simulink model "Balloon_Animation"  (R2020a)
settings: Solver=VariableStepAuto  StartTime=0.0  StopTime=100  RelTol=1e-3
libraries: vrlib x3, simulink x2, visionsinks x1
settings Model: Creator=Jeffrey  LastModifiedBy=seanchai

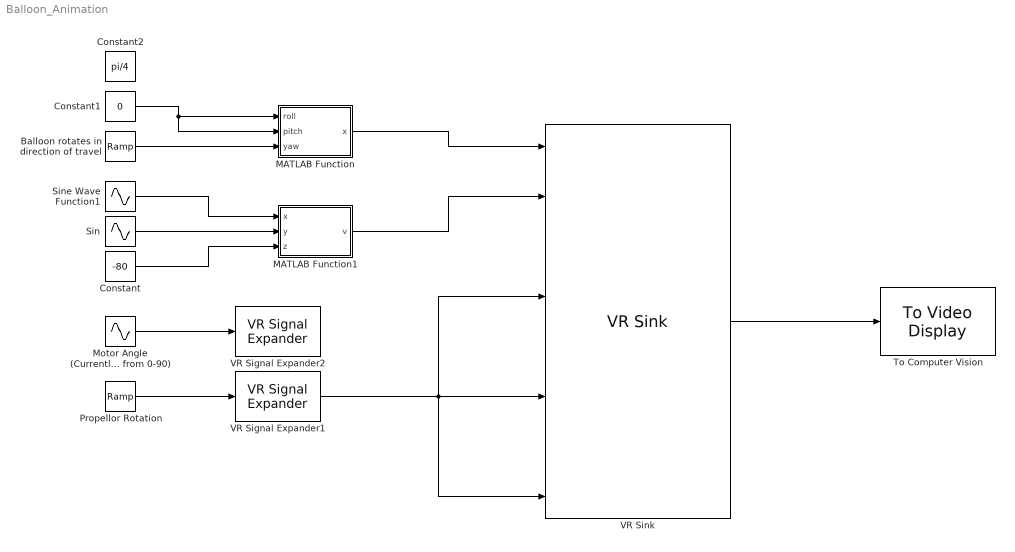
== system Balloon_Animation ==
  Balloon rotates in direction of travel : simulink/Sources/Ramp  slope=2*pi/100  start=0  InitialOutput=0
  Constant : Constant  Value=-80
  Constant1 : Constant  Value=0
  Constant2 : Constant  Value=pi/4
  MATLAB Function : MATLAB Function  TreatAsAtomicUnit=on
  MATLAB Function1 : MATLAB Function  TreatAsAtomicUnit=on
  Motor Angle (Currently rotating from 0-90) : Sin  Amplitude=pi/4  Bias=pi/4  Frequency=1/5  SampleTime=0
  Propellor Rotation : simulink/Sources/Ramp  slope=1  start=0  InitialOutput=0
  Sin : Sin  Amplitude=-20  Bias=+20  Frequency=2*pi/100  Phase=pi/2  SampleTime=0
  Sine Wave Function1 : Sin  Amplitude=20  Frequency=2*pi/100  SampleTime=0
  To Computer Vision : visionsinks/To Video Display  windowSizeMode=Normal  openAtMdlStart=on  fullScreen=off  videoWindowX=603  videoWindowY=111  saveWindowSize=off  videoWindowWidth=640  videoWindowHeight=400  inputColorFormat=RGB  inputType=Obsolete  imagePorts=One multidimensional signal  OutputDevice=On-screen video monitor  dataOrg=Column-major  isWindowOpen=off
  VR Signal Expander1 : vrlib/VR Signal Expander  outwidth=4  outidx=[4]
  VR Signal Expander2 : vrlib/VR Signal Expander  outwidth=4  outidx=[4]
  VR Sink : vrlib/VR Sink  InstantiateOnLoad=on  SampleTime=0.1  ViewEnable=on  RemoteChange=off  RemoteView=off  FieldsWritten=Airship.rotation.4.1.1.double#Airship.translation.3.1.1.double#Motor001_0001.rotation.4.1.1.double#Prop001_0001.rotation.4.1.1.double#Motor002_0001.rotation.4.1.1.double#Prop002_0001.rotation.4.1.1.double#Motor003_0001.rotation.4.1.1.double#Prop003_0001.rotation.4.1.1.double  WorldFileName=Open_Box.wrl  AutoView=on  VideoDimensions=[400 640]  AllowVariableSize=off  FigureProperties="{'Position', 'Name', 'Viewpoint', 'CameraBound', 'CameraDirection', 'CameraPosition', 'CameraUpVector', 'ZoomFactor', 'Antialiasing', 'Headlight', 'Lighting', 'NavPanel', 'Sound', 'StatusBar', 'Stereo3D', 'Stereo3DCameraOffset', 'Stereo3DHIT', 'ToolBar', 'Textures', 'Transparency', 'Triad', 'Wireframe', 'NavZones', 'NavMode', 'NavSpeed', 'CaptureFileFormat', 'CaptureFileName', 'Record2DCompressMethod', 'Record2DCompressQuality', 'Record2D', 'Record2DFileName', 'Record2DFPS'; [4.5500000000000000e+02   3.4800000000000000e+02   6.4000000000000000e+02   4.0000000000000000e+02], '', 'SensorCam2', 'on', [0.0000000000000000e+00   0.0000000000000000e+00  -1.0000000000000000e+00], [0.0000000000000000e+00   0.0000000000000000e+00   0.0000000000000000e+00], [0.0000000000000000e+00   1.0000000000000000e+00   0.0000000000000000e+00], [1.0000000000000000e+00], 'off', 'on', 'on', 'none', 'on', 'off', 'off', [1.0000000149011612e-01], [0.0000000000000000e+00], 'off', 'on', 'on', 'none', 'off', 'off', 'fly', 'normal', 'tif', '%f_anim_%n.tif', 'auto', [7.5000000000000000e+01], 'off', '***video***', 'auto'}"
  wires:
  Propellor Rotation/1 -> VR Signal Expander1/1
  Motor Angle (Currently rotating from 0-90)/1 -> VR Signal Expander2/1
  Sine Wave Function1/1 -> MATLAB Function1/1(x)
  VR Sink/1 -> To Computer Vision/1
  Sin/1 -> MATLAB Function1/2(y)
  Constant/1 -> MATLAB Function1/3(z)
  MATLAB Function/1(x) -> VR Sink/1
  MATLAB Function1/1(v) -> VR Sink/2
  VR Signal Expander1/1 -> VR Sink/4, VR Sink/6, VR Sink/8
  Constant1/1 -> MATLAB Function/1(roll), MATLAB Function/2(pitch)
  Balloon rotates in direction of travel/1 -> MATLAB Function/3(yaw)

== matlab function Balloon_Animation/MATLAB Function ==
  data: roll input; x output; pitch input; yaw input
function x = fcn(roll,pitch,yaw) %local pitch and roll
a = -roll;
b = -pitch;
c = yaw;

T_roll = [ 1, 0      , 0    ;
         0, cos(a) , sin(a) ;
         0, -sin(a), cos(a) ];
     
T_pitch = [cos(b),0,-sin(b) ;
        0     ,1,0       ;
        sin(b),0,cos(b)  ];
    
T_yaw = [cos(c) ,sin(c),0;
        -sin(c),cos(c),0;
        0      ,0     ,1];


T_BE = T_roll * T_pitch * T_yaw;
        
        
v = rotationMatrixToVector (T_BE^-1);

x = [v(1),v(3),v(2), norm(v)];

== matlab function Balloon_Animation/MATLAB Function1 ==
  data: x input; v output; y input; z input
function v = fcn(x,y,z)

v = [x , -z, y]
